simulink model "PID_cosimulation"  (R2016b)
settings: Solver=VariableStepAuto  StartTime=0.0  StopTime=10.0  RelTol=1e-3
libraries: simulink_extras x2, modelsimlib x1
settings Model: Creator=Ege  LastModifiedBy=Ege

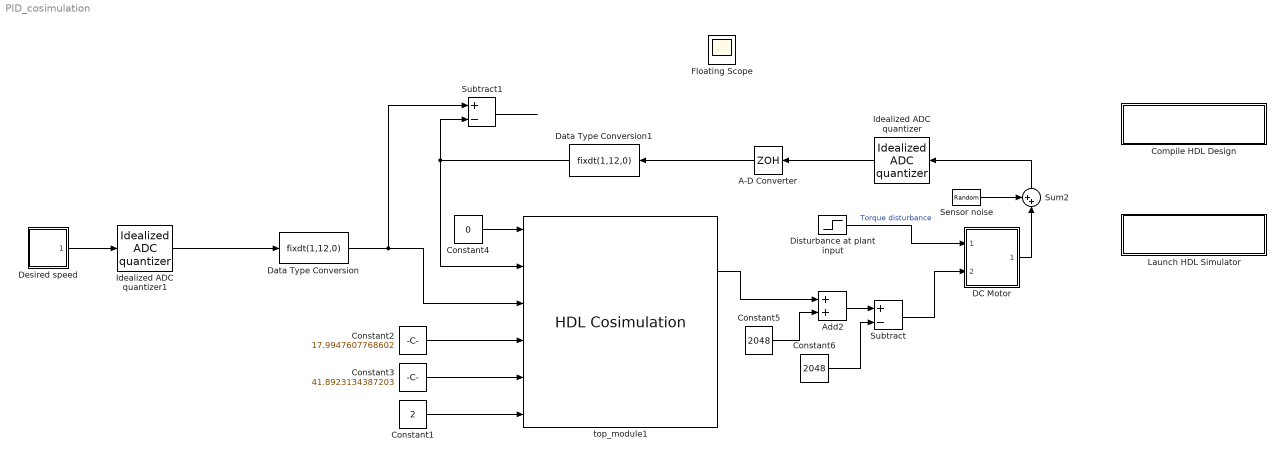
== system PID_cosimulation ==
  " Disturbance at plant input" : Step  Time=5  After=0.2  SampleTime=0
  A-D Converter : ZeroOrderHold  SampleTime=0.02
  Add2 : Sum  AccumDataTypeStr=fixdt(0,12,0)  OutDataTypeStr=double
  Compile HDL Design : Subsystem
      settings: OpenFcn=eval('compile_hdl_design_top_module');
      mask Display: disp(['Double-Click to' char(10) 'compile HDL files'])
  Constant1 : Constant  Value=2  OutDataTypeStr=fixdt(1,32,18)
  Constant2 : Constant  Value=17.9947607768602  OutDataTypeStr=fixdt(1,32,18, 'DataTypeOverride', 'Off')
  Constant3 : Constant  Value=41.8923134387203  OutDataTypeStr=fixdt(1,32,18)
  Constant4 : Constant  Value=0  OutDataTypeStr=fixdt(0,1,0, 'DataTypeOverride', 'Off')
  Constant5 : Constant  Value=2048  OutDataTypeStr=fixdt(0,12,0)
  Constant6 : Constant  Value=2048  OutDataTypeStr=double
  DC Motor : Subsystem  mask(DC Motor){b=0.1, J=0.01, K=0.01, R=1, L=0.5}
      mask prompts: b "Damping:"; J "Inertia:"; K "Back EMF:"; R "Resistance:"; L "Inductance:"
      mask help: An ideal model of a DC Motor
      mask Help: This is <b>more elaborate<b> help.
      mask Display: image(imread('dcmotor.jpg'))
  Data Type Conversion : DataTypeConversion  OutDataTypeStr=fixdt(1,12,0)
  Data Type Conversion1 : DataTypeConversion  OutDataTypeStr=fixdt(1,12,0)
  Desired speed : Subsystem
  Floating Scope : Scope
      settings: Floating=on
  Idealized ADC quantizer : simulink_extras/Additional Discrete/Idealized ADC quantizer  NumberOfConverterBits=12  Vmin=-5  Vmax=5  OutputDataType=int16  OutputNegativeValues=on
  Idealized ADC quantizer1 : simulink_extras/Additional Discrete/Idealized ADC quantizer  NumberOfConverterBits=12  Vmin=-5  Vmax=5  OutputDataType=int16  OutputNegativeValues=on
  Launch HDL Simulator : Subsystem
      settings: OpenFcn=eval('launch_hdl_simulator_top_module');
      mask Display: disp(['Double-Click to' char(10) 'launch HDL simulator'])
  Sensor noise : RandomNumber  Variance=0.05  SampleTime=0.02
  Subtract : Sum  Inputs=+-  AccumDataTypeStr=double  OutDataTypeStr=double
  Subtract1 : Sum  Inputs=+-  AccumDataTypeStr=double  OutDataTypeStr=double
  Sum2 : Sum  Inputs=++|
  top_module1 : modelsimlib/HDL Cosimulation  PortPaths=/top_module/i_reset;/top_module/i_feedback;/top_module/i_reference;/top_module/i_kp;/top_module/i_ki;/top_module/i_kd;/top_module/o_output;/top_module/o_overflow  PortModes=[1 1 1 1 1 1 2 2 ]  PortTimes=[-1,-1,-1,-1,-1,-1,0.001,1]  PortSigns=[-1 -1 -1 -1 -1 -1 -1 -1 ]  PortFracLengths=[0,0,0,0,0,0,0,0]  CommLocal=on  CommSharedMemory=off  CommPortNumber=61934  CommShowInfo=on  ClockModes=[]  ClockTimes=[]  TclPreSimCommand=|  TclPostSimCommand=|  TimingMode=s  TimingScaleFactor=0.0001  idxCellArray={'UNUSED_VAR'}  CosimBypass=Full Simulation  AllowDirectFeedthrough=on  ProductName=EDA Simulator Link MQ  RunAutoTimescale=off  HdlClocks=/top_module/i_clk 10 ns;/top_module/i_adc_clk 10 ns;  PreRunTime=0  PreRunTimeUnit=ns
      TclPreSimCommand=|
      | force /top_module/i_clk 0 0 ns, 1 1 ns -repeat 2 ns;
      | force /top_module/i_adc_clk 0 0 ns, 1 5 ns -repeat 10 ns;
      TclPostSimCommand=|
      | noforce /top_module/i_adc_clk;
      | noforce /top_module/i_clk;
      | puts "done";
  wires:
  Idealized ADC quantizer/1 -> A-D Converter/1
  Desired speed/1(Speed) -> Idealized ADC quantizer1/1
  Constant1/1 -> top_module1/6
  Constant2/1 -> top_module1/4
  A-D Converter/1 -> Data Type Conversion1/1
  Idealized ADC quantizer1/1 -> Data Type Conversion/1
  top_module1/1 -> Add2/1
  Constant5/1 -> Add2/2
  Add2/1 -> Subtract/1
  Subtract/1 -> DC Motor/2(Voltage)
  Constant6/1 -> Subtract/2
  Subtract1/1 -> ?
  Data Type Conversion/1 -> Subtract1/1, top_module1/3
  Data Type Conversion1/1 -> top_module1/2, Subtract1/2
  " Disturbance at plant input"/1 -> DC Motor/1(Torque)  "Torque disturbance"
  Sensor noise/1 -> Sum2/1
  DC Motor/1(Speed) -> Sum2/2
  Sum2/1 -> Idealized ADC quantizer/1
  Constant3/1 -> top_module1/5
  Constant4/1 -> top_module1/1

== system PID_cosimulation/Compile HDL Design ==

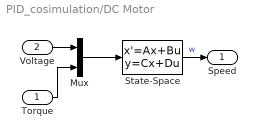
== system PID_cosimulation/DC Motor ==
  Torque : Inport
  Voltage : Inport  Port=2
  Mux : Mux  Inputs=2
  State-Space : StateSpace  A=[-b/J K/J; -K/L -R/L]  B=[0 -1/J; 1/L 0]  C=[1 0]  D=[0 0]  X0=0
  Speed : Outport
  wires:
  Mux/1 -> State-Space/1
  Voltage/1 -> Mux/1
  State-Space/1 -> Speed/1  "w"
  Torque/1 -> Mux/2

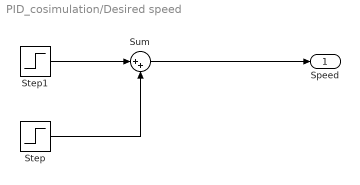
== system PID_cosimulation/Desired speed ==
  Step : Step  Time=7  After=-4  SampleTime=0.02
  Step1 : Step  After=2  SampleTime=0.02
  Sum : Sum  Inputs=|++
  Speed : Outport
  wires:
  Step/1 -> Sum/2
  Step1/1 -> Sum/1
  Sum/1 -> Speed/1

== system PID_cosimulation/Launch HDL Simulator ==
